simulink model "Dinamica_del_rollio_1gdl"  (Simulink 7.8)
settings: Solver=ode45  StartTime=0.0  StopTime=2  RelTol=1e-3
settings Model: Creator=Adriano  LastModifiedBy=Adriano

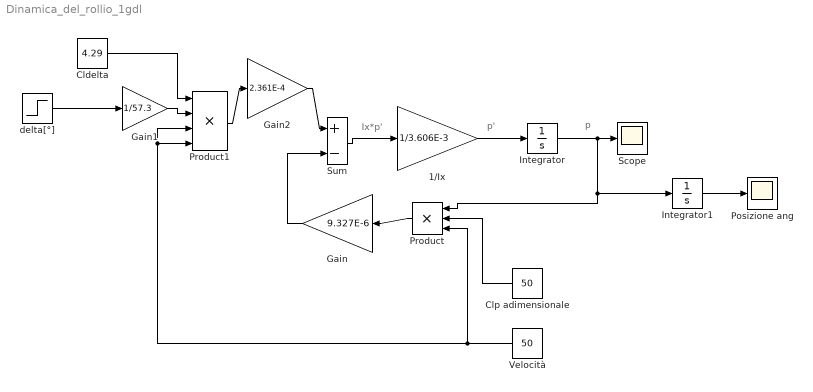
== system Dinamica_del_rollio_1gdl ==
  note: Ix*p'
  note: p'
  note: p
  1/Ix : Gain  Gain=1/3.606E-3
  Cldelta : Constant  Value=4.29
  Clp adimensionale : Constant  Value=50
  Gain : Gain  Gain=9.327E-6
  Gain1 : Gain  Gain=1/57.3
  Gain2 : Gain  Gain=2.361E-4
  Integrator : Integrator
  Integrator1 : Integrator
  Posizione ang : Scope
      settings: TimeRange=10  YMin=0  YMax=7
  Product : Product  Inputs=3  RndMeth=Zero
  Product1 : Product  Inputs=4  RndMeth=Zero
  Scope : Scope
      settings: TimeRange=10  YMin=0  YMax=7
  Sum : Sum  Inputs=+-
  Velocità : Constant  Value=50
  delta[°] : Step  After=9  SampleTime=0
  wires:
  Sum/1 -> 1/Ix/1
  1/Ix/1 -> Integrator/1
  Integrator/1 -> Scope/1, Product/1, Integrator1/1
  Clp adimensionale/1 -> Product/2
  Velocità/1 -> Product/3, Product1/3, Product1/4
  delta[°]/1 -> Gain1/1
  Gain1/1 -> Product1/2
  Cldelta/1 -> Product1/1
  Product1/1 -> Gain2/1
  Gain2/1 -> Sum/1
  Gain/1 -> Sum/2
  Product/1 -> Gain/1
  Integrator1/1 -> Posizione ang/1
